simulink model "pv_mppt_boost_converter"  (R2019a)
settings: Solver=VariableStepAuto  StartTime=0.0  StopTime=10.0  RelTol=1e-3
libraries: powerlib x9, re_lib x1, powerlib_meascontrol x1
settings Model: Creator=vinic  LastModifiedBy=vinic

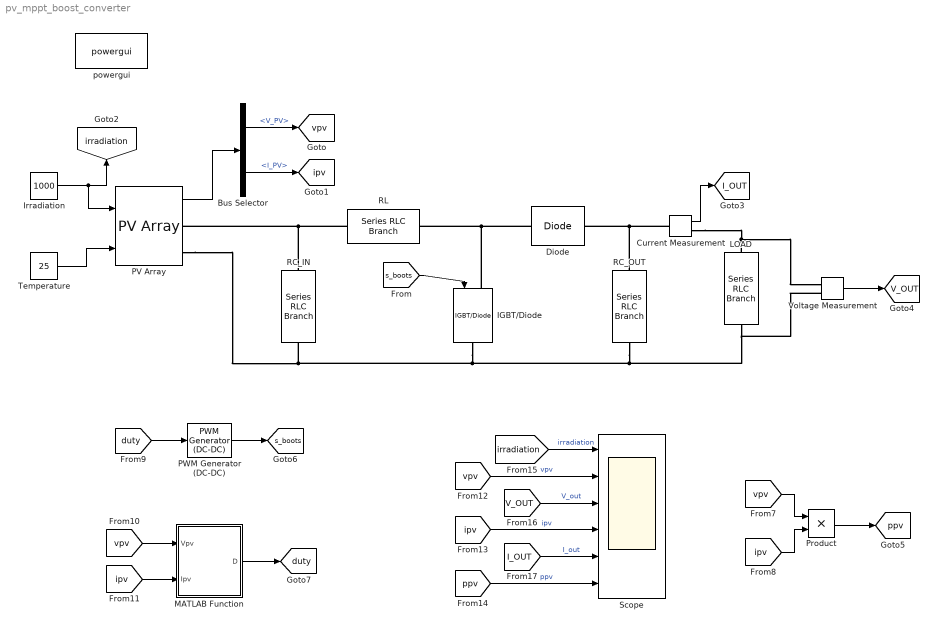
== system pv_mppt_boost_converter ==
  Bus Selector : BusSelector  OutputSignals=V_PV,I_PV
  Current Measurement : powerlib/Measurements/Current Measurement  PhasorSimulation=off  OutputType=Complex  PSBequivalent=0
      settings: SourceProductName=Simscape Electrical
  Diode : powerlib/Power Electronics/Diode  Ron=0.001  Lon=0  Vf=0.8  IC=0  UseSnubber=0  Rs=500  Cs=250e-9  Measurements=off
      settings: SourceProductName=Simscape Electrical
  IGBT/Diode : powerlib/Power Electronics/IGBT//Diode  Ron=1e-3  Rs=1e5  Cs=inf  Measurements=off
      settings: SourceProductName=Simscape Electrical
  Irradiation : Constant  Value=1000
  LOAD : powerlib/Elements/Series RLC Branch  LConnTagsString=__new0  RConnTagsString=__new0  BranchType=R  Resistance=100  Inductance=1e-3  SetiL0=off  InitialCurrent=0  Capacitance=3300e-6  Setx0=off  InitialVoltage=0  Measurements=None
      settings: SourceProductName=Simscape Electrical
  MATLAB Function : MATLAB Function  TreatAsAtomicUnit=on
  PV Array : re_lib/Solar/PV Array  Npar=5  Nser=1  PlotType=array @ 1000 W/m2 & specified temperatures  S_vec="[ 1000  500  100 ]"  Temp_C_vec="[ 45 25  ]"  ModuleName=1Soltech 1STH-215-P  PlotWhenSelected=off  Pm=213.15  Ncell=60  Voc=36.3  Isc=7.84  Vm=29  Im=7.35  beta_Voc_pc=-0.36099  alpha_Isc_pc=0.102  beta_Voc=-0.13104  alpha_Isc=0.007997  IL=7.8649  I0=2.9259e-10  nI=0.98117  Rsh=313.3991  Rs=0.39383  BAL=off  Tc=1e-6  Tfilter=5e-5
      settings: SourceProductName=Simscape Electrical
  PWM Generator (DC-DC) : powerlib_meascontrol/Pulse & Signal Generators/PWM Generator (DC-DC)  Fsw=5000  Ts=10e-6
      settings: SourceProductName=Simscape Electrical
  Product : Product
  RC_IN : powerlib/Elements/Series RLC Branch  LConnTagsString=__new0  RConnTagsString=__new0  BranchType=RC  Resistance=1e-4  Inductance=1e-3  SetiL0=off  InitialCurrent=0  Capacitance=100e-6  Setx0=off  InitialVoltage=0  Measurements=None
      settings: SourceProductName=Simscape Electrical
  RC_OUT : powerlib/Elements/Series RLC Branch  LConnTagsString=__new0  RConnTagsString=__new0  BranchType=RC  Resistance=1e-4  Inductance=1e-3  SetiL0=off  InitialCurrent=0  Capacitance=3300e-6  Setx0=off  InitialVoltage=0  Measurements=None
      settings: SourceProductName=Simscape Electrical
  RL : powerlib/Elements/Series RLC Branch  LConnTagsString=__new0  RConnTagsString=__new0  BranchType=RL  Resistance=1e-4  Inductance=1e-3  SetiL0=off  InitialCurrent=0  Capacitance=1e-6  Setx0=off  InitialVoltage=0  Measurements=None
      settings: SourceProductName=Simscape Electrical
  Scope : Scope  NumInputPorts=6
  Temperature : Constant  Value=25
  Voltage Measurement : powerlib/Measurements/Voltage Measurement  PhasorSimulation=off  OutputType=Complex  PSBequivalent=0
      settings: SourceProductName=Simscape Electrical
  powergui : powerlib/powergui  Priority=1  SimulationMode=Continuous  SampleTime=50e-6  frequency=60  Iterations=50  frequencyindice=0  Pbase=100e6  ErrMax=1e-4  UnitsV=kV  UnitsW=MW  buscounter=0  FunctionMessages=off  echomessages=off  EnableUseOfTLC=off  CurrentSourceSwitches=off  DisableSnubberDevices=off  DisableRonSwitches=off  DisableVfSwitches=off  DisplayEquations=off  AutomaticDiscreteSolvers=off  SolverType=Tustin/Backward Euler (TBE)  Interpol=off  ExternalGateDelay=off  methode=off  Ts=100  x0status=blocks  SPID=on  SwTol=0  HookPort=off  NonlinearTolerance=0  nMaxIteration=15  ContinueOnMaxIteration=off  RestoreLinks=warning  ResistiveCurrentMeasurement=off  Frange=[0:2:500]  Ylog=off  Xlog=on  ShowGrid=off  save=off  variable=ZData  structure=0  ZoomFFT=off  StartTime=0.0  cycles=1  DisplayStyle=1  fundamental=60  FreqAxis=off  MaxFrequency=1000  frequencyindicesteady=1  RmsSteady=1  display=off
      settings: SourceProductName=Simscape Electrical
  tag scope: I_OUT=global, V_OUT=global, duty=global, ipv=global, irradiation=global, ppv=global, s_boots=global, vpv=global
  wires:
  PV Array/1 -> Bus Selector/1
  Bus Selector/1 -> [vpv]  "<V_PV>"
  Bus Selector/2 -> [ipv]  "<I_PV>"
  Irradiation/1 -> [irradiation], PV Array/1
  Temperature/1 -> PV Array/2
  [s_boots] -> IGBT/Diode/1
  Voltage Measurement/1 -> [V_OUT]
  Current Measurement/1 -> [I_OUT]
  [irradiation] -> Scope/1  "irradiation"
  [vpv] -> Scope/2  "vpv"
  [V_OUT] -> Scope/3  "V_out"
  [ipv] -> Scope/4  "ipv"
  [I_OUT] -> Scope/5  "I_out"
  [ppv] -> Scope/6  "ppv"
  [vpv] -> Product/1
  [ipv] -> Product/2
  Product/1 -> [ppv]
  PWM Generator (DC-DC)/1 -> [s_boots]
  [duty] -> PWM Generator (DC-DC)/1
  MATLAB Function/1(D) -> [duty]
  [vpv] -> MATLAB Function/1(Vpv)
  [ipv] -> MATLAB Function/2(Ipv)
  connections:
  PV Array/RConn2 -- Voltage Measurement/LConn2 -- LOAD/RConn1 -- RC_OUT/RConn1 -- IGBT/Diode/RConn1 -- RC_IN/RConn1
  RC_IN/LConn1 -- RL/RConn1 -- PV Array/RConn1
  IGBT/Diode/LConn1 -- Diode/LConn1 -- RL/LConn1
  LOAD/LConn1 -- Current Measurement/RConn1 -- Voltage Measurement/LConn1
  RC_OUT/LConn1 -- Current Measurement/LConn1 -- Diode/RConn1

== matlab function pv_mppt_boost_converter/MATLAB Function ==
  settings: updateMethod=DISCRETE
  data: Vpv input; D output; Ipv input
function D = PandO(Vpv,Ipv)

persistent Dprev Pprev Vprev

if isempty(Dprev)
    Dprev=0.7;
    Vprev=190;
    Pprev=2000;
end


deltaD = 125e-6;

%Calculate measured array power
Ppv=Vpv*Ipv;

%Increase or decrease duty cycle based on conditions
if(Ppv-Pprev) ~= 0
    if(Ppv-Pprev)>0
        if(Vpv-Vprev)>0
            D = Dprev-deltaD;
        else
            D = Dprev+deltaD;
        end
    else
        if(Vpv-Vprev)>0
            D = Dprev+deltaD;
        else
            D = Dprev-deltaD;
        end
    end
else
    D = Dprev;
end

%Update internal values
Dprev = D;
Vprev = Vpv;
Pprev = Ppv;
